simulink model "mech_clutch"  (Simulink 7.1)
settings: Solver=ode45  StartTime=0.0  StopTime=10.0  RelTol=1e-3  AbsTol=1e-6
PreLoadFcn:
  | load clutchparam.mat
values from neighbouring files (symbols this model uses):
  R = y([30:p],2)./y([30:p],1)    [mech_car_handling_sweep.m]    (also in mech_flexible_beamelement.m = [1  0  0; mech_sceng_init.m = 5; mech_toroid_setup.m = 10)
undefined symbols (not defined in the file or in its folder): be, bv, Ie, Iv, muk, mus
libraries: mblibv1 x12
Description:
  | Clutch Mechanism
  | 
  | This model demonstrates a clutch mechanism using traditional Simulink blocks (in red) and using SimMechanics blocks (in blue). The model using SimMechanics blocks is simpler than the one using pure Simulink blocks.
settings Model: Creator=gwood  LastModifiedBy=batserve  ExtModeAutoUpdateStatusClock=off
settings DataIOCC: SignalLoggingName=logsOut
settings OptimizationCC: BooleanDataType=off  InlineInvariantSignals=on
settings DebuggingCC: AlgebraicLoopMsg=none  SaveWithParameterizedLinksMsg=none  CheckExecutionContextPreStartOutputMsg=on  CheckExecutionContextRuntimeOutputMsg=on  SignalResolutionControl=TryResolveAllWithWarning  SolverPrmCheckMsg=none  MultiTaskDSMMsg=warning  MultiTaskCondExecSysMsg=none  SigSpecEnsureSampleTimeMsg=none  StrictBusMsg=None
settings HardwareCC: TargetBitPerLong=64  TargetEndianess=LittleEndian  TargetWordSize=64  TargetHWDeviceType=MATLAB Host  ProdEqTarget=off
settings RTWCC: SystemTargetFile=rsim.tlc  TemplateMakefile=rsim_default_tmf  Description=Rapid Simulation Target  ProcessScript=rsim_make_rtw_hook  IncludeERTFirstTime=on
settings RSimTargetCC: TargetFcnLib=ansi_tfl_tmw.mat  TargetFunctionLibrary=ANSI_C  IsPILTarget=off  EnableShiftOperators=on  PortableWordSizes=off

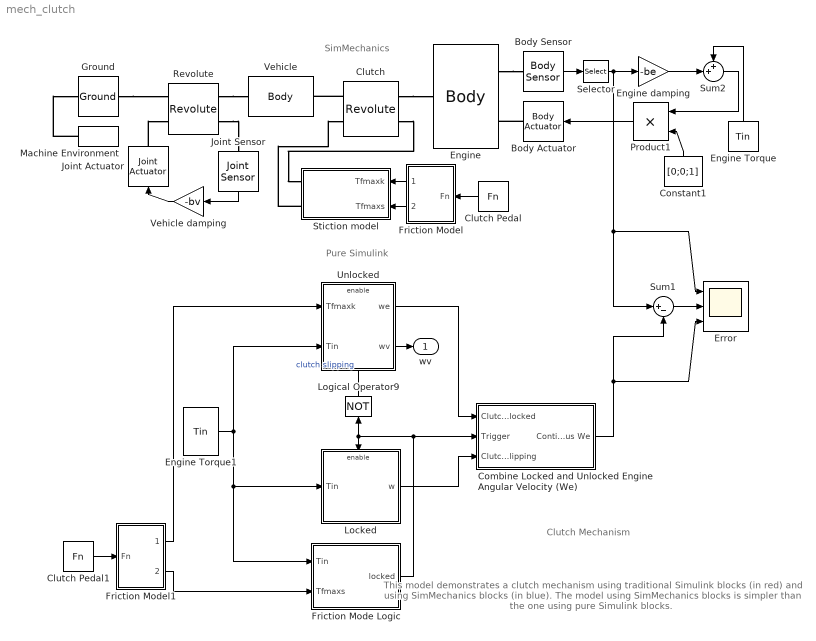
== system mech_clutch ==
  note: Clutch Mechanism
  note: Pure Simulink
  note: SimMechanics
  note: This model demonstrates a clutch mechanism using traditional
      | Simulink blocks (in red) and using SimMechanics blocks (in blue).
      | The model using SimMechanics blocks is simpler than the one
      | using pure Simulink blocks.
  Body Actuator : mblibv1/Sensors &  Actuators/Body Actuator  Orientation=left  DialogController=MECH.DynMechDlgSource  SystemSampleTime=-1  PhysicalDomain=Mechanical  PortType=blob  ActuationStyle=Force  AngleUnits=deg  ArcVelocityUnits=deg/s  ArcAccelerationUnits=deg/s^2  CoordPositionUnits=m  VelocityUnits=m/s  AccelerationUnits=m/s^2  ForceUnits=N  TorqueUnits=N-m  ActiveIO=on  Width=3  DialogClass=MechanicalActuatorBlock  ReferenceFrame=Absolute (World)  Angle=off  CoordPosition=on  Force=off  Torque=on
  Body Sensor : mblibv1/Sensors &  Actuators/Body Sensor  DialogController=MECH.DynMechDlgSource  SystemSampleTime=-1  PhysicalDomain=Mechanical  PortType=blob  Muxed=on  Pose=off  Angle=on  AngleUnits=deg  ArcVelocity=on  ArcVelocityUnits=rad/s  ArcAcceleration=off  ArcAccelerationUnits=deg/s^2  CoordPosition=off  CoordPositionUnits=m  Velocity=off  VelocityUnits=m/s  Acceleration=off  AccelerationUnits=m/s^2  Quaternion=on  QuaternionDT=off  QuaternionDDT=off  QuaternionUnits=off  OutputVector=[ 3 ]  ActiveIO=on  Width=3  DialogClass=MechanicalSensorBlock  ReferenceFrame=Absolute (World)
  Clutch : mblibv1/Joints/Revolute  Orientation=left  DialogController=MECH.DynMechDlgSource  PhysicalDomain=mechanical  SubClassName=Unknown  LeftPortType=blob  RightPortType=blob  LConnTagsString=__newl0|SA1  RConnTagsString=__newr0|SA1  NumSAPorts=2  CutJoint=off  MarkAsCut=off  Primitives=revolute  PrimitiveProps=R1$WORLD$[0 0 1]$revolute  DialogClass=JointBlock  R1Axis=[0 0 1]
  Clutch Pedal : FromWorkspace  Orientation=left  VariableName=Fn  SampleTime=0
  Clutch Pedal1 : FromWorkspace  VariableName=Fn  SampleTime=0
  Combine Locked and Unlocked Engine Angular Velocity (We) : Subsystem
  Constant1 : Constant  Orientation=up  Value=[0;0;1]  OutDataType=sfix(16)  OutScaling=2^0
  Engine : mblibv1/Bodies/Body  DialogController=MECH.DynMechDlgSource  PhysicalDomain=mechanical  SubClassName=Unknown  LeftPortType=workingframe  RightPortType=workingframe  LConnTagsString=CS1  RConnTagsString=CS2|CS3  DialogClass=MechanicalBodyBlock  Mass=1  MassUnits=kg  InertiaUnits=kg*m^2  Inertia=diag([0;0;Ie])  Shape=Cylinder  ShapeDims=[1 1]  ShapeUnits=m  ShapeUse=false  Density=1  DensityUnits=kg/m^3  DensityUse=false  GraphicsMode=1  BodyColor=[0.5 0.5 0.5]  GraphicsObj=[]  AttachedToCS=1  CG=Left$CG$[0 0 0]$WORLD$WORLD$m$[0 0 0]$Euler X-Y-Z$deg$WORLD$false  WorkingFrames=Left$CS1$[0 0 0]$CG$CG$m$[0 0 0]$Euler X-Y-Z$deg$WORLD$true#Right$CS2$[0 0 0]$CG$CG$m$[0 0 0]$Euler X-Y-Z$deg$WORLD$true#Right$CS3$[0 0 0]$CG$CG$m$[0 0 0]$Euler X-Y-Z$deg$WORLD$true  CGPos=[0 0 0]  CGRot=[0 0 0]  CS0Pos=[]  CS0Rot=[]  CS1Pos=[0 0 0]  CS1Rot=[0 0 0]  CS2Pos=[0 0 0]  CS2Rot=[0 0 0]  CS3Pos=[0 0 0]  CS3Rot=[0 0 0]  CS4Pos=[]  CS4Rot=[]  CS5Pos=[]  CS5Rot=[]  CS6Pos=[]  CS6Rot=[]  CS7Pos=[]  CS7Rot=[]  CS8Pos=[]  CS8Rot=[]  CS9Pos=[]  CS9Rot=[]  CS10Pos=[]  CS10Rot=[]  CS11Pos=[]  CS11Rot=[]  CS12Pos=[]  CS12Rot=[]  CS13Pos=[]  CS13Rot=[]  CS14Pos=[]  CS14Rot=[]  CS15Pos=[]  CS15Rot=[]  CS16Pos=[]  CS16Rot=[]  CS17Pos=[]  CS17Rot=[]  CS18Pos=[]  CS18Rot=[]  CS19Pos=[]  CS19Rot=[]  CS20Pos=[]  CS20Rot=[]
  Engine Torque : FromWorkspace  Orientation=up  VariableName=Tin  SampleTime=0
  Engine Torque1 : FromWorkspace  VariableName=Tin  SampleTime=0
  Engine damping : Gain  Gain=-be  ParameterDataType=sfix(16)  ParameterScaling=2^0  OutDataType=sfix(16)  OutScaling=2^0  SaturateOnIntegerOverflow=on  OutDataTypeStr=Inherit: Same as input  ParamDataTypeStr=Inherit: Same as input
  Error : Scope  NumInputPorts=3
      settings: TimeRange=10  YMin=0~-1e-014~0  YMax=0.8~5e-014~0.8
  Friction Model : Subsystem  Orientation=left
  Friction Model1 : Subsystem
  Friction Mode Logic : Subsystem
      mask Display: plot([-3 1 1 3 -1 -1],[-1 -1 1 1 1 -1],-4,-5,4,5)
  Ground : mblibv1/Bodies/Ground  DialogController=MECH.DynMechDlgSource  SystemSampleTime=-1  LeftPortType=env  RightPortType=workingframe  PhysicalDomain=Mechanical  DialogClass=GroundBlock  CoordPosition=[0 0 0]  CoordPositionUnits=m  StateVectorMgrId=-1  MachineId=[0 0]  ShowEnvPort=on
  Joint Actuator : mblibv1/Sensors &  Actuators/Joint Actuator  Orientation=up  DialogController=MECH.DynMechDlgSource  SystemSampleTime=-1  PhysicalDomain=Mechanical  PortType=blob  ActuationStyle=Force  AngleUnits=deg  ArcVelocityUnits=deg/s  ArcAccelerationUnits=deg/s^2  CoordPositionUnits=m  VelocityUnits=m/s  AccelerationUnits=m/s^2  ForceUnits=N  TorqueUnits=N-m  ActiveIO=on  Width=1  DialogClass=MechanicalActuatorBlock  Primitive=R1  ReferenceFrame=Absolute (INERTIAL)
  Joint Sensor : mblibv1/Sensors &  Actuators/Joint Sensor  Orientation=down  DialogController=MECH.DynMechDlgSource  SystemSampleTime=-1  PhysicalDomain=Mechanical  PortType=blob  Muxed=on  Pose=off  Angle=off  AngleUnits=deg  ArcVelocity=on  ArcVelocityUnits=rad/s  ArcAcceleration=off  ArcAccelerationUnits=deg/s^2  CoordPosition=on  CoordPositionUnits=m  Velocity=off  VelocityUnits=m/s  Acceleration=off  AccelerationUnits=m/s^2  Quaternion=on  QuaternionDT=off  QuaternionDDT=off  QuaternionUnits=off  OutputVector=[ 1 ]  ActiveIO=on  Width=1  DialogClass=MechanicalSensorBlock  Primitive=R1  Force=off  ForceUnits=N  Torque=off  TorqueUnits=N-m  ReferenceFrame=Absolute (INERTIAL)  ReactionSensedSide=Base  ReactionReferenceFrame=Absolute (World)  ReactionForce=off  ReactionForceUnits=N  ReactionMoment=off  ReactionMomentUnits=N-m
  Locked : Subsystem  TreatAsAtomicUnit=on
      mask Display: plot(-1,-6,6,12,[0 3],[3 3],[3 1 1 3], [1 1 5 5],[2 4 4 2],[4 4 2 2],[4 5],[3 3])
  Logical Operator9 : Logic  Orientation=up  Operator=NOT  Inputs=1
      mask Display: plot(0, -.25, 2., .5, [0 2 0 0], [-.5 0 .5 -.5],.2*cos(0:.1:2*pi)+2.2, .1*sin(0:.1:2*pi))
  Machine Environment : mblibv1/Bodies/Machine Environment  Tag=Factory ground  Orientation=left  DialogController=MECH.DialogSource  SystemSampleTime=-1  PortType=env  PhysicalDomain=Mechanical  DialogTemplateClass=MECH.MachineEnvironment  SyncWhenCopied=off  Gravity=[0 0 0]  GravityUnits=m/s^2  GravityAsSignal=off  Dimensionality=3D Only  AnalysisType=Forward dynamics  LinearAssemblyTolerance=1e-3  LinearAssemblyToleranceUnits=m  AngularAssemblyTolerance=1e-3  AngularAssemblyToleranceUnits=rad  ConstraintSolverType=Stabilizing  ConstraintRelTolerance=1e-4  ConstraintAbsTolerance=1e-4  UseRobustSingularityHandling=off  RedundancyAnalysisToleranceType=Automatically select tolerance  RedundancyAnalysisTolerance=1e-14  StatePerturbationType=Fixed  PerturbationSize=1e-5  VisualizeMachine=on
  Product1 : Product  Orientation=left  OutDataType=sfix(16)  OutScaling=2^0  SaturateOnIntegerOverflow=on  RndMeth=Zero  InputSameDT=on  OutDataTypeStr=Inherit: Same as first input
  Revolute : mblibv1/Joints/Revolute  DialogController=MECH.DynMechDlgSource  PhysicalDomain=mechanical  SubClassName=Unknown  LeftPortType=blob  RightPortType=blob  LConnTagsString=__newl0|SA1  RConnTagsString=__newr0|SA1  NumSAPorts=2  CutJoint=off  MarkAsCut=off  Primitives=revolute  PrimitiveProps=R1$WORLD$[0 0 1]$revolute  DialogClass=JointBlock  R1Axis=[0 0 1]
  Selector : Selector  InputPortWidth=3  IndexOptions=Index vector (dialog)  Indices=3  OutputSizes=1
  Stiction model : Subsystem  Orientation=left
  Sum1 : Sum  Inputs=|+-  OutDataType=sfix(16)  OutScaling=2^0  SaturateOnIntegerOverflow=on  InputSameDT=on  OutDataTypeStr=Inherit: Same as first input
  Sum2 : Sum  Inputs=++|  OutDataType=sfix(16)  OutScaling=2^0  SaturateOnIntegerOverflow=on  InputSameDT=on  OutDataTypeStr=Inherit: Same as first input
  Unlocked : Subsystem  TreatAsAtomicUnit=on
      mask Display: plot(-1,-2,6,8,[0 3],[3 3],[3 1 1 3], [1 1 5 5],[2 4 4 2],[4 4 2 2],[4 5],[3 3])
  Vehicle : mblibv1/Bodies/Body  DialogController=MECH.DynMechDlgSource  PhysicalDomain=mechanical  SubClassName=Unknown  LeftPortType=workingframe  RightPortType=workingframe  LConnTagsString=CS1  RConnTagsString=CS2  DialogClass=MechanicalBodyBlock  Mass=0  MassUnits=kg  InertiaUnits=kg*m^2  Inertia=diag([0;0;Iv])  Shape=Cylinder  ShapeDims=[1 1]  ShapeUnits=m  ShapeUse=false  Density=1  DensityUnits=kg/m^3  DensityUse=false  GraphicsMode=1  BodyColor=[0.5 0.5 0.5]  GraphicsObj=[]  AttachedToCS=1  CG=Left$CG$[0 0 0]$WORLD$WORLD$m$[0 0 0]$Euler X-Y-Z$deg$WORLD$false  WorkingFrames=Left$CS1$[0 0 0]$CG$CG$m$[0 0 0]$Euler X-Y-Z$deg$WORLD$true#Right$CS2$[0 0 0]$CG$CG$m$[0 0 0]$Euler X-Y-Z$deg$WORLD$true  CGPos=[0 0 0]  CGRot=[0 0 0]  CS0Pos=[]  CS0Rot=[]  CS1Pos=[0 0 0]  CS1Rot=[0 0 0]  CS2Pos=[0 0 0]  CS2Rot=[0 0 0]  CS3Pos=[]  CS3Rot=[]  CS4Pos=[]  CS4Rot=[]  CS5Pos=[]  CS5Rot=[]  CS6Pos=[]  CS6Rot=[]  CS7Pos=[]  CS7Rot=[]  CS8Pos=[]  CS8Rot=[]  CS9Pos=[]  CS9Rot=[]  CS10Pos=[]  CS10Rot=[]  CS11Pos=[]  CS11Rot=[]  CS12Pos=[]  CS12Rot=[]  CS13Pos=[]  CS13Rot=[]  CS14Pos=[]  CS14Rot=[]  CS15Pos=[]  CS15Rot=[]  CS16Pos=[]  CS16Rot=[]  CS17Pos=[]  CS17Rot=[]  CS18Pos=[]  CS18Rot=[]  CS19Pos=[]  CS19Rot=[]  CS20Pos=[]  CS20Rot=[]
  Vehicle damping : Gain  Orientation=left  Gain=-bv  ParameterDataType=sfix(16)  ParameterScaling=2^0  OutDataType=sfix(16)  OutScaling=2^0  SaturateOnIntegerOverflow=on  OutDataTypeStr=Inherit: Same as input  ParamDataTypeStr=Inherit: Same as input
  wv : Outport  OutDataType=sfix(16)  OutScaling=2^0  InitialOutput=0
  wires:
  Joint Sensor/1 -> Vehicle damping/1
  Vehicle damping/1 -> Joint Actuator/1
  Body Sensor/1 -> Selector/1
  Product1/1 -> Body Actuator/1
  Clutch Pedal/1 -> Friction Model/1(Fn)
  Friction Model/1(Tfmaxk) -> Stiction model/1(Tfmaxk)
  Friction Model/2(Tfmaxs) -> Stiction model/2(Tfmaxs)
  Selector/1 -> Engine damping/1, Error/1, Sum1/1
  Engine damping/1 -> Sum2/2
  Sum2/1 -> Product1/1
  Constant1/1 -> Product1/2
  Engine Torque1/1 -> Unlocked/2(Tin), Friction Mode Logic/1(Tin), Locked/1(Tin)
  Friction Model1/1(Tfmaxk) -> Unlocked/1(Tfmaxk)
  Unlocked/2(wv) -> wv/1
  Locked/1(w) -> Combine Locked and Unlocked Engine Angular Velocity (We)/3(Clutch slipping)
  Logical Operator9/1 -> Unlocked/Enable  "clutch slipping"
  Friction Model1/2(Tfmaxs) -> Friction Mode Logic/2(Tfmaxs)
  Clutch Pedal1/1 -> Friction Model1/1(Fn)
  Engine Torque/1 -> Sum2/1
  Unlocked/1(we) -> Combine Locked and Unlocked Engine Angular Velocity (We)/1(Clutch locked)
  Friction Mode Logic/1(locked) -> Combine Locked and Unlocked Engine Angular Velocity (We)/2(Trigger), Locked/Enable, Logical Operator9/1
  Combine Locked and Unlocked Engine Angular Velocity (We)/1(Continuous We) -> Error/3, Sum1/2
  Sum1/1 -> Error/2
  connections:
  Revolute/RConn1 -- Vehicle/LConn1
  Revolute/RConn2 -- Joint Sensor/LConn1
  Joint Actuator/RConn1 -- Revolute/LConn2
  Engine/RConn1 -- Body Sensor/LConn1
  Body Actuator/RConn1 -- Engine/RConn2
  Clutch/RConn1 -- Vehicle/RConn1
  Clutch/LConn1 -- Engine/LConn1
  Clutch/LConn2 -- Stiction model/RConn1
  Stiction model/RConn2 -- Clutch/RConn2
  Ground/RConn1 -- Revolute/LConn1
  Machine Environment/RConn1 -- Ground/LConn1

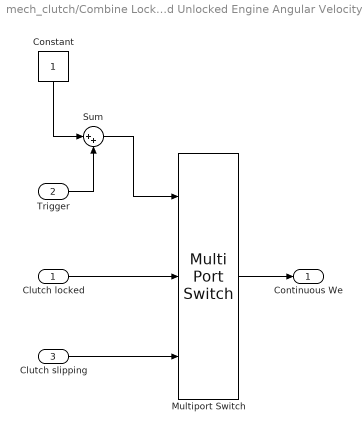
== system mech_clutch/Combine Locked and Unlocked Engine Angular Velocity (We) ==
  Clutch locked : Inport  OutDataType=sfix(16)  OutScaling=2^0
  Trigger : Inport  Port=2  OutDataType=sfix(16)  OutScaling=2^0
  Clutch slipping : Inport  Port=3  OutDataType=sfix(16)  OutScaling=2^0
  Constant : Constant  Orientation=down  OutDataType=sfix(16)  OutScaling=2^0
  Multiport Switch : MultiPortSwitch  Inputs=2  SaturateOnIntegerOverflow=on  InputSameDT=on
  Sum : Sum  Inputs=|++  OutDataType=sfix(16)  OutScaling=2^0  SaturateOnIntegerOverflow=on  InputSameDT=on  OutDataTypeStr=Inherit: Same as first input
  Continuous We : Outport  OutDataType=sfix(16)  OutScaling=2^0
  wires:
  Constant/1 -> Sum/1
  Trigger/1 -> Sum/2
  Multiport Switch/1 -> Continuous We/1
  Clutch locked/1 -> Multiport Switch/2
  Clutch slipping/1 -> Multiport Switch/3
  Sum/1 -> Multiport Switch/1

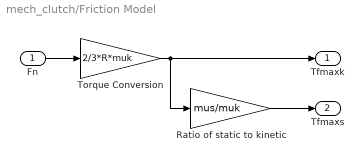
== system mech_clutch/Friction Model ==
  Fn : Inport  OutDataType=sfix(16)  OutScaling=2^0
  Ratio of static to kinetic : Gain  Gain=mus/muk  ParameterDataType=sfix(16)  ParameterScaling=2^0  OutDataType=sfix(16)  OutScaling=2^0  SaturateOnIntegerOverflow=on  OutDataTypeStr=Inherit: Same as input  ParamDataTypeStr=Inherit: Same as input
  Torque Conversion : Gain  Gain=2/3*R*muk  ParameterDataType=sfix(16)  ParameterScaling=2^0  OutDataType=sfix(16)  OutScaling=2^0  SaturateOnIntegerOverflow=on  OutDataTypeStr=Inherit: Same as input  ParamDataTypeStr=Inherit: Same as input
  Tfmaxk : Outport  OutDataType=sfix(16)  OutScaling=2^0  InitialOutput=0
  Tfmaxs : Outport  Port=2  OutDataType=sfix(16)  OutScaling=2^0  InitialOutput=0
  wires:
  Torque Conversion/1 -> Tfmaxk/1, Ratio of static to kinetic/1
  Fn/1 -> Torque Conversion/1
  Ratio of static to kinetic/1 -> Tfmaxs/1

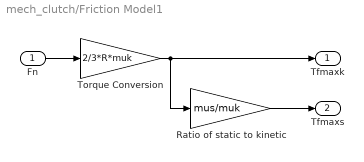
== system mech_clutch/Friction Model1 ==
  Fn : Inport  OutDataType=sfix(16)  OutScaling=2^0
  Ratio of static to kinetic : Gain  Gain=mus/muk  ParameterDataType=sfix(16)  ParameterScaling=2^0  OutDataType=sfix(16)  OutScaling=2^0  SaturateOnIntegerOverflow=on  OutDataTypeStr=Inherit: Same as input  ParamDataTypeStr=Inherit: Same as input
  Torque Conversion : Gain  Gain=2/3*R*muk  ParameterDataType=sfix(16)  ParameterScaling=2^0  OutDataType=sfix(16)  OutScaling=2^0  SaturateOnIntegerOverflow=on  OutDataTypeStr=Inherit: Same as input  ParamDataTypeStr=Inherit: Same as input
  Tfmaxk : Outport  OutDataType=sfix(16)  OutScaling=2^0  InitialOutput=0
  Tfmaxs : Outport  Port=2  OutDataType=sfix(16)  OutScaling=2^0  InitialOutput=0
  wires:
  Ratio of static to kinetic/1 -> Tfmaxs/1
  Fn/1 -> Torque Conversion/1
  Torque Conversion/1 -> Ratio of static to kinetic/1, Tfmaxk/1

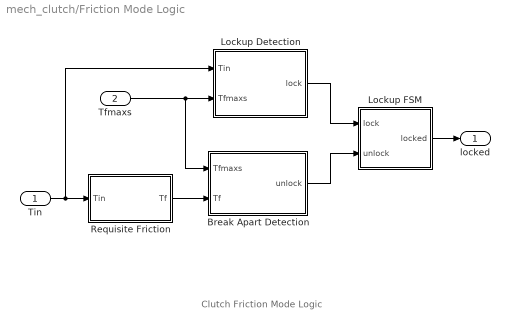
== system mech_clutch/Friction Mode Logic ==
  note: Clutch Friction Mode Logic
  Tin : Inport  OutDataType=sfix(16)  OutScaling=2^0
  Tfmaxs : Inport  Port=2  OutDataType=sfix(16)  OutScaling=2^0
  Break Apart Detection : Subsystem
  Lockup Detection : Subsystem
  Lockup FSM : Subsystem
  Requisite Friction : Subsystem
  locked : Outport  OutDataType=sfix(16)  OutScaling=2^0  InitialOutput=0
  wires:
  Lockup FSM/1(locked) -> locked/1
  Lockup Detection/1(lock) -> Lockup FSM/1(lock)
  Break Apart Detection/1(unlock) -> Lockup FSM/2(unlock)
  Requisite Friction/1(Tf) -> Break Apart Detection/2(Tf)
  Tfmaxs/1 -> Break Apart Detection/1(Tfmaxs), Lockup Detection/2(Tfmaxs)
  Tin/1 -> Requisite Friction/1(Tin), Lockup Detection/1(Tin)

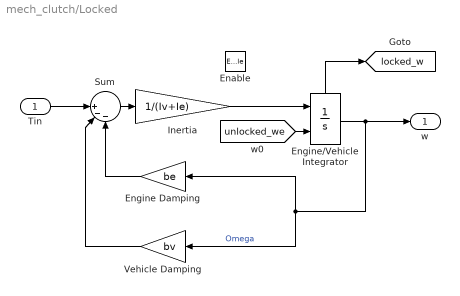
== system mech_clutch/Locked ==
  Tin : Inport  OutDataType=sfix(16)  OutScaling=2^0
  Enable : EnablePort  StatesWhenEnabling=reset
  Engine Damping : Gain  Orientation=left  Gain=be  ParameterDataType=sfix(16)  ParameterScaling=2^0  OutDataType=sfix(16)  OutScaling=2^0  SaturateOnIntegerOverflow=on  OutDataTypeStr=Inherit: Same as input  ParamDataTypeStr=Inherit: Same as input
  Engine/Vehicle Integrator : Integrator  InitialConditionSource=external  ShowStatePort=on
  Inertia : Gain  Gain=1/(Iv+Ie)  ParameterDataType=sfix(16)  ParameterScaling=2^0  OutDataType=sfix(16)  OutScaling=2^0  SaturateOnIntegerOverflow=on  OutDataTypeStr=Inherit: Same as input  ParamDataTypeStr=Inherit: Same as input
  Sum : Sum  Inputs=||+--  OutDataType=sfix(16)  OutScaling=2^0  SaturateOnIntegerOverflow=on  InputSameDT=on  OutDataTypeStr=Inherit: Same as first input
  Vehicle Damping : Gain  Orientation=left  Gain=bv  ParameterDataType=sfix(16)  ParameterScaling=2^0  OutDataType=sfix(16)  OutScaling=2^0  SaturateOnIntegerOverflow=on  OutDataTypeStr=Inherit: Same as input  ParamDataTypeStr=Inherit: Same as input
  w : Outport  OutDataType=sfix(16)  OutScaling=2^0  InitialOutput=0
  tag scope: locked_w=global
  wires:
  Vehicle Damping/1 -> Sum/2
  Inertia/1 -> Engine/Vehicle Integrator/1
  Engine Damping/1 -> Sum/3
  Engine/Vehicle Integrator/1 -> Vehicle Damping/1, Engine Damping/1, w/1  "Omega"
  Tin/1 -> Sum/1
  Sum/1 -> Inertia/1
  Engine/Vehicle Integrator/State -> [locked_w]
  [unlocked_we] -> Engine/Vehicle Integrator/2

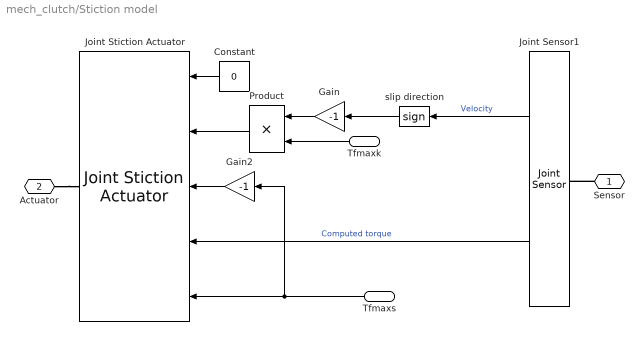
== system mech_clutch/Stiction model ==
  Tfmaxk : Inport  Orientation=left  OutDataType=sfix(16)  OutScaling=2^0
  Tfmaxs : Inport  Orientation=left  Port=2  OutDataType=sfix(16)  OutScaling=2^0
  Constant : Constant  Orientation=left  Value=0  OutDataType=sfix(16)  OutScaling=2^0
  Gain : Gain  Orientation=left  Gain=-1  ParameterDataType=sfix(16)  ParameterScaling=2^0  OutDataType=sfix(16)  OutScaling=2^0  SaturateOnIntegerOverflow=on  OutDataTypeStr=Inherit: Same as input  ParamDataTypeStr=Inherit: Same as input
  Gain2 : Gain  Orientation=left  Gain=-1  ParameterDataType=sfix(16)  ParameterScaling=2^0  OutDataType=sfix(16)  OutScaling=2^0  SaturateOnIntegerOverflow=on  OutDataTypeStr=Inherit: Same as input  ParamDataTypeStr=Inherit: Same as input
  Joint Sensor1 : mblibv1/Sensors &  Actuators/Joint Sensor  Orientation=left  DialogController=MECH.DynMechDlgSource  SystemSampleTime=-1  PhysicalDomain=Mechanical  PortType=blob  Muxed=off  Pose=off  Angle=off  AngleUnits=deg  ArcVelocity=on  ArcVelocityUnits=rad/s  ArcAcceleration=off  ArcAccelerationUnits=deg/s^2  CoordPosition=on  CoordPositionUnits=m  Velocity=off  VelocityUnits=m/s  Acceleration=off  AccelerationUnits=m/s^2  Quaternion=on  QuaternionDT=off  QuaternionDDT=off  QuaternionUnits=off  OutputVector=[ 1 1 ]  ActiveIO=on  Width=2  DialogClass=MechanicalSensorBlock  Primitive=R1  Force=off  ForceUnits=N  Torque=on  TorqueUnits=N-m  ReferenceFrame=Absolute (INERTIAL)  ReactionSensedSide=Base  ReactionReferenceFrame=Absolute (World)  ReactionForce=off  ReactionForceUnits=N  ReactionMoment=off  ReactionMomentUnits=N-m
  Joint Stiction Actuator : mblibv1/Sensors &  Actuators/Joint Stiction Actuator  Orientation=left  DialogController=MECH.DynMechDlgSource  SystemSampleTime=-1  PhysicalDomain=Mechanical  PortType=blob  ActuationStyle=Force  AngleUnits=deg  ArcVelocityUnits=deg/s  ArcAccelerationUnits=deg/s^2  CoordPositionUnits=m  VelocityUnits=m/s  AccelerationUnits=m/s^2  ForceUnits=N  TorqueUnits=N-m  ActiveIO=on  Width=5  DialogClass=EventActuatorBlock  Primitive=R1  FrictionalForceUnits=N  ExternalForceUnits=N  FrictionalTorqueUnits=N-m  ExternalTorqueUnits=N-m  LockingTolerance=1e-3
  Product : Product  Orientation=left  OutDataType=sfix(16)  OutScaling=2^0  SaturateOnIntegerOverflow=on  RndMeth=Zero  InputSameDT=on  OutDataTypeStr=Inherit: Same as first input
  slip direction : Signum  Orientation=left
  Sensor : PMIOPort  Orientation=left  Port=1  Side=Right
  Actuator : PMIOPort  Port=2  Side=Right
  wires:
  Joint Sensor1/1 -> slip direction/1  "Velocity"
  Product/1 -> Joint Stiction Actuator/2
  Gain/1 -> Product/1
  slip direction/1 -> Gain/1
  Gain2/1 -> Joint Stiction Actuator/3
  Tfmaxk/1 -> Product/2
  Joint Sensor1/2 -> Joint Stiction Actuator/4  "Computed torque"
  Constant/1 -> Joint Stiction Actuator/1
  Tfmaxs/1 -> Gain2/1, Joint Stiction Actuator/5
  connections:
  Sensor/RConn1 -- Joint Sensor1/LConn1
  Actuator/RConn1 -- Joint Stiction Actuator/RConn1

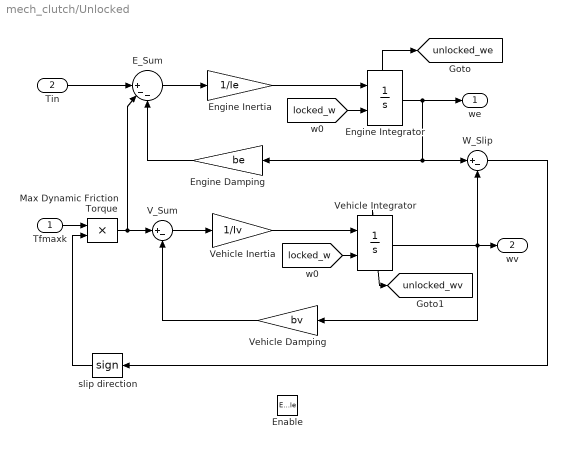
== system mech_clutch/Unlocked ==
  Tfmaxk : Inport  OutDataType=sfix(16)  OutScaling=2^0
  Tin : Inport  Port=2  OutDataType=sfix(16)  OutScaling=2^0
  Enable : EnablePort  StatesWhenEnabling=reset
  E_Sum : Sum  Inputs=||+--  OutDataType=sfix(16)  OutScaling=2^0  SaturateOnIntegerOverflow=on  InputSameDT=on  OutDataTypeStr=Inherit: Same as first input
  Engine Damping : Gain  Orientation=left  Gain=be  ParameterDataType=sfix(16)  ParameterScaling=2^0  OutDataType=sfix(16)  OutScaling=2^0  SaturateOnIntegerOverflow=on  OutDataTypeStr=Inherit: Same as input  ParamDataTypeStr=Inherit: Same as input
  Engine Inertia : Gain  Gain=1/Ie  ParameterDataType=sfix(16)  ParameterScaling=2^0  OutDataType=sfix(16)  OutScaling=2^0  SaturateOnIntegerOverflow=on  OutDataTypeStr=Inherit: Same as input  ParamDataTypeStr=Inherit: Same as input
  Engine Integrator : Integrator  InitialConditionSource=external  ShowStatePort=on
  Max Dynamic Friction Torque : Product  OutDataType=sfix(16)  OutScaling=2^0  SaturateOnIntegerOverflow=on  RndMeth=Zero  InputSameDT=on  OutDataTypeStr=Inherit: Same as first input
  V_Sum : Sum  Inputs=|+-  OutDataType=sfix(16)  OutScaling=2^0  SaturateOnIntegerOverflow=on  InputSameDT=on  OutDataTypeStr=Inherit: Same as first input
  Vehicle Damping : Gain  Orientation=left  Gain=bv  ParameterDataType=sfix(16)  ParameterScaling=2^0  OutDataType=sfix(16)  OutScaling=2^0  SaturateOnIntegerOverflow=on  OutDataTypeStr=Inherit: Same as input  ParamDataTypeStr=Inherit: Same as input
  Vehicle Inertia : Gain  Gain=1/Iv  ParameterDataType=sfix(16)  ParameterScaling=2^0  OutDataType=sfix(16)  OutScaling=2^0  SaturateOnIntegerOverflow=on  OutDataTypeStr=Inherit: Same as input  ParamDataTypeStr=Inherit: Same as input
  Vehicle Integrator : Integrator  InitialConditionSource=external  ShowStatePort=on
  W_Slip : Sum  Inputs=|+-  OutDataType=sfix(16)  OutScaling=2^0  SaturateOnIntegerOverflow=on  InputSameDT=on  OutDataTypeStr=Inherit: Same as first input
  slip direction : Signum  Orientation=left
  we : Outport  OutDataType=sfix(16)  OutScaling=2^0  InitialOutput=0
  wv : Outport  Port=2  OutDataType=sfix(16)  OutScaling=2^0  InitialOutput=0
  tag scope: unlocked_we=global, unlocked_wv=global
  wires:
  Vehicle Integrator/1 -> W_Slip/2, wv/1, Vehicle Damping/1
  Vehicle Inertia/1 -> Vehicle Integrator/1
  [locked_w] -> Vehicle Integrator/2
  Vehicle Integrator/State -> [unlocked_wv]
  Tin/1 -> E_Sum/1
  [locked_w] -> Engine Integrator/2
  Engine Integrator/1 -> W_Slip/1, Engine Damping/1, we/1
  Engine Damping/1 -> E_Sum/3
  E_Sum/1 -> Engine Inertia/1
  Engine Inertia/1 -> Engine Integrator/1
  Engine Integrator/State -> [unlocked_we]
  W_Slip/1 -> slip direction/1
  slip direction/1 -> Max Dynamic Friction Torque/2
  Tfmaxk/1 -> Max Dynamic Friction Torque/1
  Max Dynamic Friction Torque/1 -> E_Sum/2, V_Sum/1
  Vehicle Damping/1 -> V_Sum/2
  V_Sum/1 -> Vehicle Inertia/1

== system mech_clutch/Friction Mode Logic/Break Apart Detection ==
  Tfmaxs : Inport  OutDataType=sfix(16)  OutScaling=2^0
  Tf : Inport  Port=2  OutDataType=sfix(16)  OutScaling=2^0
  Abs : Abs  SaturateOnIntegerOverflow=on
  Relational Operator : RelationalOperator  InputSameDT=on
  unlock : Outport  OutDataType=sfix(16)  OutScaling=2^0  InitialOutput=0
  wires:
  Tfmaxs/1 -> Relational Operator/2
  Abs/1 -> Relational Operator/1
  Relational Operator/1 -> unlock/1
  Tf/1 -> Abs/1

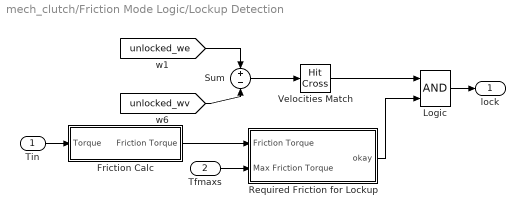
== system mech_clutch/Friction Mode Logic/Lockup Detection ==
  Tin : Inport  OutDataType=sfix(16)  OutScaling=2^0
  Tfmaxs : Inport  Port=2  OutDataType=sfix(16)  OutScaling=2^0
  Friction Calc : Subsystem
  Logic : Logic
  Required Friction for Lockup : Subsystem
  Sum : Sum  Inputs=+-  OutDataType=sfix(16)  OutScaling=2^0  SaturateOnIntegerOverflow=on  InputSameDT=on  OutDataTypeStr=Inherit: Same as first input
  Velocities Match : HitCross
  lock : Outport  OutDataType=sfix(16)  OutScaling=2^0  InitialOutput=0
  wires:
  Tin/1 -> Friction Calc/1(Torque)
  Sum/1 -> Velocities Match/1
  [unlocked_wv] -> Sum/2
  [unlocked_we] -> Sum/1
  Required Friction for Lockup/1(okay) -> Logic/2
  Logic/1 -> lock/1
  Velocities Match/1 -> Logic/1
  Tfmaxs/1 -> Required Friction for Lockup/2(Max Friction Torque)
  Friction Calc/1(Friction Torque) -> Required Friction for Lockup/1(Friction Torque)

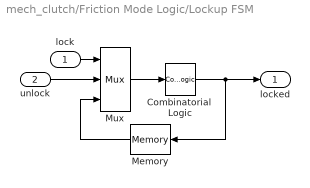
== system mech_clutch/Friction Mode Logic/Lockup FSM ==
  lock : Inport  OutDataType=sfix(16)  OutScaling=2^0
  unlock : Inport  Port=2  OutDataType=sfix(16)  OutScaling=2^0
  Combinatorial  Logic : CombinatorialLogic  TruthTable=[0;1;0;0;1;1;1;0]
  Memory : Memory  Orientation=left
  Mux : Mux  Inputs=3
  locked : Outport  OutDataType=sfix(16)  OutScaling=2^0  InitialOutput=0
  wires:
  Mux/1 -> Combinatorial  Logic/1
  lock/1 -> Mux/1
  unlock/1 -> Mux/2
  Combinatorial  Logic/1 -> Memory/1, locked/1
  Memory/1 -> Mux/3

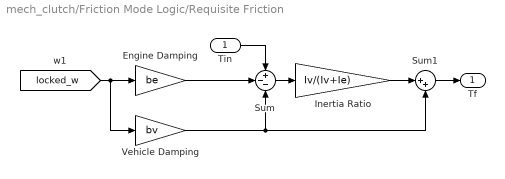
== system mech_clutch/Friction Mode Logic/Requisite Friction ==
  Tin : Inport  OutDataType=sfix(16)  OutScaling=2^0
  Engine Damping : Gain  Gain=be  ParameterDataType=sfix(16)  ParameterScaling=2^0  OutDataType=sfix(16)  OutScaling=2^0  SaturateOnIntegerOverflow=on  OutDataTypeStr=Inherit: Same as input  ParamDataTypeStr=Inherit: Same as input
  Inertia Ratio : Gain  Gain=Iv/(Iv+Ie)  ParameterDataType=sfix(16)  ParameterScaling=2^0  OutDataType=sfix(16)  OutScaling=2^0  SaturateOnIntegerOverflow=on  OutDataTypeStr=Inherit: Same as input  ParamDataTypeStr=Inherit: Same as input
  Sum : Sum  Inputs=+--  OutDataType=sfix(16)  OutScaling=2^0  SaturateOnIntegerOverflow=on  InputSameDT=on  OutDataTypeStr=Inherit: Same as first input
  Sum1 : Sum  Inputs=|++  OutDataType=sfix(16)  OutScaling=2^0  SaturateOnIntegerOverflow=on  InputSameDT=on  OutDataTypeStr=Inherit: Same as first input
  Vehicle Damping : Gain  Gain=bv  ParameterDataType=sfix(16)  ParameterScaling=2^0  OutDataType=sfix(16)  OutScaling=2^0  SaturateOnIntegerOverflow=on  OutDataTypeStr=Inherit: Same as input  ParamDataTypeStr=Inherit: Same as input
  Tf : Outport  OutDataType=sfix(16)  OutScaling=2^0  InitialOutput=0
  wires:
  Sum1/1 -> Tf/1
  Inertia Ratio/1 -> Sum1/1
  Tin/1 -> Sum/1
  Sum/1 -> Inertia Ratio/1
  Vehicle Damping/1 -> Sum1/2, Sum/3
  Engine Damping/1 -> Sum/2
  [locked_w] -> Engine Damping/1, Vehicle Damping/1

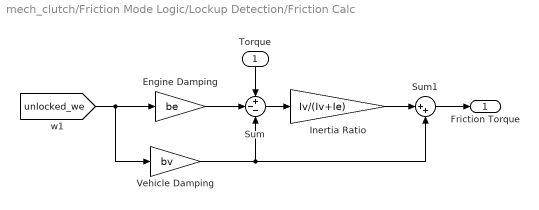
== system mech_clutch/Friction Mode Logic/Lockup Detection/Friction Calc ==
  Torque : Inport  Orientation=down  OutDataType=sfix(16)  OutScaling=2^0
  Engine Damping : Gain  Gain=be  ParameterDataType=sfix(16)  ParameterScaling=2^0  OutDataType=sfix(16)  OutScaling=2^0  SaturateOnIntegerOverflow=on  OutDataTypeStr=Inherit: Same as input  ParamDataTypeStr=Inherit: Same as input
  Inertia Ratio : Gain  Gain=Iv/(Iv+Ie)  ParameterDataType=sfix(16)  ParameterScaling=2^0  OutDataType=sfix(16)  OutScaling=2^0  SaturateOnIntegerOverflow=on  OutDataTypeStr=Inherit: Same as input  ParamDataTypeStr=Inherit: Same as input
  Sum : Sum  Inputs=+--  OutDataType=sfix(16)  OutScaling=2^0  SaturateOnIntegerOverflow=on  InputSameDT=on  OutDataTypeStr=Inherit: Same as first input
  Sum1 : Sum  Inputs=|++  OutDataType=sfix(16)  OutScaling=2^0  SaturateOnIntegerOverflow=on  InputSameDT=on  OutDataTypeStr=Inherit: Same as first input
  Vehicle Damping : Gain  Gain=bv  ParameterDataType=sfix(16)  ParameterScaling=2^0  OutDataType=sfix(16)  OutScaling=2^0  SaturateOnIntegerOverflow=on  OutDataTypeStr=Inherit: Same as input  ParamDataTypeStr=Inherit: Same as input
  Friction Torque : Outport  OutDataType=sfix(16)  OutScaling=2^0  InitialOutput=0
  wires:
  Sum1/1 -> Friction Torque/1
  Inertia Ratio/1 -> Sum1/1
  Torque/1 -> Sum/1
  Sum/1 -> Inertia Ratio/1
  Engine Damping/1 -> Sum/2
  Vehicle Damping/1 -> Sum/3, Sum1/2
  [unlocked_we] -> Vehicle Damping/1, Engine Damping/1

== system mech_clutch/Friction Mode Logic/Lockup Detection/Required Friction for Lockup ==
  Friction Torque : Inport  OutDataType=sfix(16)  OutScaling=2^0
  Max Friction Torque : Inport  Port=2  OutDataType=sfix(16)  OutScaling=2^0
  Abs : Abs  SaturateOnIntegerOverflow=on
  Relational Operator : RelationalOperator  Operator=<=  InputSameDT=on
  okay : Outport  OutDataType=sfix(16)  OutScaling=2^0  InitialOutput=0
  wires:
  Max Friction Torque/1 -> Relational Operator/2
  Abs/1 -> Relational Operator/1
  Relational Operator/1 -> okay/1
  Friction Torque/1 -> Abs/1
